simulink model "RB_KAIROS_BaseOnly"  (R2020b)
settings: Solver=ode4  StartTime=0.0  StopTime=t_end  FixedStep=Ts  RelTol=1e-3
values from neighbouring files (symbols this model uses):
  am = 0.3    [RB_KAIROS_ImpControl_OpSpace_BaseOnly.m]
  am_r = 0.3    [RB_KAIROS_ImpControl_OpSpace_BaseOnly.m]
  Jv = [1 0 0; 0 1 0; 0 0 0; 0 0 0; 0 0 0; 0 0 1;]    [RB_KAIROS_ImpControl_OpSpace_BaseOnly.m]
  Kc = diag(5*[1000,1000,0,0,0,1000])    [RB_KAIROS_ImpControl_OpSpace_BaseOnly.m]
  model_sample_time = 0.001    [RB_KAIROS_ImpControl_OpSpace_BaseOnly.m]
  q_dot_0 = zeros(10,1)    [RB_KAIROS_ImpControl_OpSpace_BaseOnly.m]
  T_i = T_W_V    [RB_KAIROS_ImpControl_OpSpace_BaseOnly.m]
  tau_ext = [0 0 0]    [RB_KAIROS_ImpControl_OpSpace_BaseOnly.m]
  v_SMU = 10    [RB_KAIROS_ImpControl_OpSpace_BaseOnly.m]
  vm = 0.6    [RB_KAIROS_ImpControl_OpSpace_BaseOnly.m]
  vm_r = 0.6    [RB_KAIROS_ImpControl_OpSpace_BaseOnly.m]
undefined symbols (not defined in the file or in its folder): DiscIntNeverNeededParam, magnitude, q_0, T_f
libraries: simulink x4, utils x4, transformations_lib x1
(part 2 of 16)

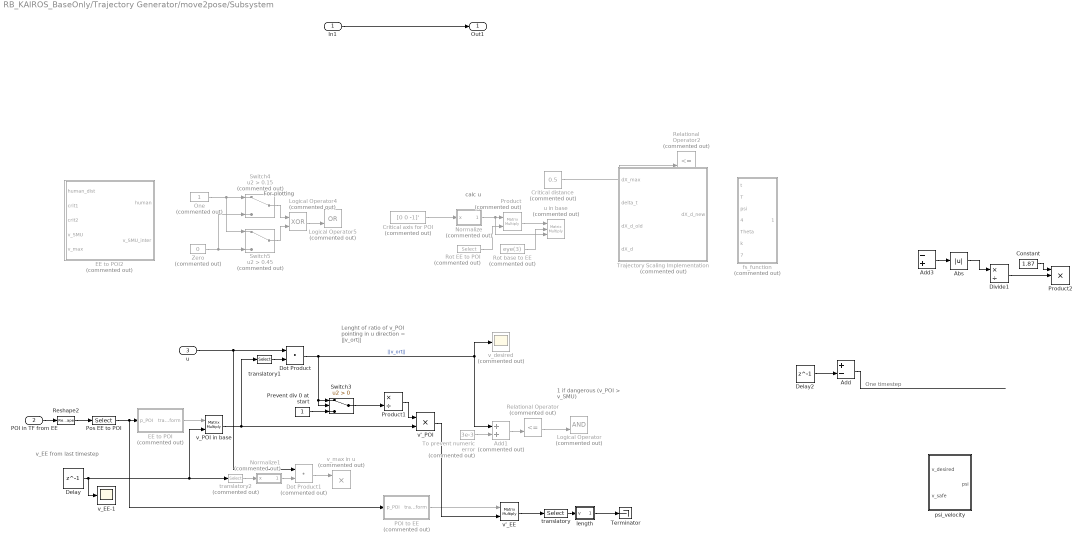
== system RB_KAIROS_BaseOnly/Trajectory Generator/move2pose/Subsystem ==
  note: calc u
  note: For plotting
  note: v_EE from last timestep
  note: 1 if dangerous
      | (v_POI > v_SMU)
  note: Lenght of ratio of v_POI
      | pointing in u direction
      | = ||v_ort||
  note: One timestep
  In1 : Inport
  POI in TF from EE : Inport  Port=2
  u : Inport  Port=3
  Abs : Abs
  Add : Sum  Inputs=+-
  Add1 : Sum  Commented=on
  Add3 : Sum  Inputs=-+
  Constant : Constant  Value=1.87
  Critical axis for POI : Constant  Commented=on  Value=[0 0 -1]'
  Critical distance : Constant  Commented=on  Value=0.5
  Delay : Delay  DelayLength=1
  Delay2 : Delay  DelayLength=1
  Divide1 : Product  Inputs=*/
  Dot Product : DotProduct  InputSameDT=on  OutDataTypeStr=Inherit: Inherit via internal rule
  Dot Product1 : DotProduct  Commented=on  InputSameDT=on  OutDataTypeStr=Inherit: Inherit via internal rule
  EE to POI : MATLAB Function  Commented=on  TreatAsAtomicUnit=on
  EE to POI2 : MATLAB Function  Commented=on  TreatAsAtomicUnit=on
  Logical Operator : Logic  Commented=on  AllPortsSameDT=off  OutDataTypeStr=boolean
  Logical Operator4 : Logic  Commented=on  Operator=XOR  AllPortsSameDT=off  OutDataTypeStr=boolean
  Logical Operator5 : Logic  Commented=on  Operator=OR  AllPortsSameDT=off  OutDataTypeStr=boolean
  Normalize : Subsystem  Commented=on
  Normalize1 : Subsystem  Commented=on
  One : Constant  Commented=on
  POI to EE : MATLAB Function  Commented=on  TreatAsAtomicUnit=on
  Pos EE to POI : Selector  NumberOfDimensions=2  InputPortWidth=7  IndexOptions=Index vector (dialog),Index vector (dialog)  Indices=[1:3],[4]  OutputSizes=1
  Prevent div 0 at start : Constant
  Product : Product  Commented=on  Multiplication=Matrix(*)
  Product1 : Product  Inputs=*/
  Product2 : Product  Inputs=3
  Relational Operator : RelationalOperator  Commented=on  Operator=<=  OutDataTypeStr=boolean  RndMeth=Simplest
  Relational Operator2 : RelationalOperator  Commented=on  Operator=<=  OutDataTypeStr=boolean  RndMeth=Simplest
  Reshape2 : Reshape  OutputDimensionality=Customize  OutputDimensions=[4,4]
  Rot EE to POI : Selector  Commented=on  NumberOfDimensions=2  InputPortWidth=7  IndexOptions=Index vector (dialog),Index vector (dialog)  Indices=[1:3],[1:3]  OutputSizes=1
  Rot base to EE : Constant  Commented=on  Value=eye(3)
  Switch3 : Switch  Criteria=u2 > Threshold
  Switch4 : Switch  Commented=on  Criteria=u2 > Threshold  Threshold=0.15
  Switch5 : Switch  Commented=on  Criteria=u2 > Threshold  Threshold=0.45
  Terminator : Terminator
  To prevent numeric error : Constant  Commented=on  Value=3e-3
  Trajectory Scaling Implementation : MATLAB Function  Commented=on  TreatAsAtomicUnit=on
  Zero : Constant  Commented=on  Value=0
  fs_function : MATLAB Function  Commented=on  TreatAsAtomicUnit=on
  length : Subsystem
  psi_velocity : MATLAB Function  TreatAsAtomicUnit=on
  translatory : Selector  InputPortWidth=6  IndexOptions=Index vector (dialog)  Indices=[1:3]  OutputSizes=1
  translatory1 : Selector  InputPortWidth=6  IndexOptions=Index vector (dialog)  Indices=[1:3]  OutputSizes=1
  translatory2 : Selector  Commented=on  InputPortWidth=6  IndexOptions=Index vector (dialog)  Indices=[1:3]  OutputSizes=1
  u in base : Product  Commented=on  Inputs=3  Multiplication=Matrix(*)
  v'_EE : Product  Multiplication=Matrix(*)
  v'_POI : Product
  v_EE-1 : Scope
  v_POI in base : Product  Multiplication=Matrix(*)
  v_desired : Scope  Commented=on
  v_max in u : Product  Commented=on
  Out1 : Outport  VectorParamsAs1DForOutWhenUnconnected=off
  wires:
  In1/1 -> Out1/1
  Critical axis for POI/1 -> Normalize/1(x)
  Rot EE to POI/1 -> Product/2
  Logical Operator4/1 -> Logical Operator5/2
  Product/1 -> u in base/1
  One/1 -> Switch4/1, Switch5/1
  Zero/1 -> Switch5/3, Switch4/3
  Switch4/1 -> Logical Operator4/1
  Switch5/1 -> Logical Operator4/2
  Normalize/1(x/||x||) -> u in base/3, Product/1
  Rot base to EE/1 -> u in base/2
  Critical distance/1 -> Relational Operator2/2
  Prevent div 0 at start/1 -> Switch3/3
  translatory2/1 -> Normalize1/1(x)
  Normalize1/1(x/||x||) -> Dot Product1/2
  ? -> Logical Operator/1
  ? -> v_max in u/2
  POI to EE/1(transform) -> v'_EE/1
  Add1/1 -> Relational Operator/2
  ? -> Product1/1
  v'_EE/1 -> translatory/1
  v'_POI/1 -> v'_EE/2
  EE to POI/1(transform) -> v_POI in base/1
  translatory/1 -> length/1(v)
  ? -> Relational Operator/1
  ? -> Delay/1
  v_POI in base/1 -> v'_POI/2, translatory1/1
  Dot Product1/1 -> v_max in u/1
  Delay/1 -> v_EE-1/1, v_POI in base/2, translatory2/1
  Dot Product/1 -> v_desired/1, Add1/1, Switch3/2, Switch3/1  "||v_ort||"
  translatory1/1 -> Dot Product/2
  Switch3/1 -> Product1/2
  Pos EE to POI/1 -> POI to EE/1(p_POI), EE to POI/1(p_POI)
  Reshape2/1 -> Pos EE to POI/1
  u/1 -> Dot Product/1, Dot Product1/1
  POI in TF from EE/1 -> Reshape2/1
  To prevent numeric error/1 -> Add1/2
  Product1/1 -> v'_POI/1
  length/1(|v|) -> Terminator/1
  Relational Operator/1 -> Logical Operator/2
  Delay2/1 -> Add/2
  ? -> Add/1
  ? -> Delay2/1
  Add/1 -> ?
  Abs/1 -> Divide1/1
  Constant/1 -> Product2/1
  Divide1/1 -> Product2/2
  Add3/1 -> Abs/1

== system RB_KAIROS_BaseOnly/CONTROLLER /Kinematics and Dynamics/Kinematics - error representation/Compute J_x_dot ==
  note: J_x_dot = R_D_W_aug*J_b_dot - R_D_W_aug*S(omega_d)_aug*J_b = R_D_W_aug*(J_b_dot - S(omega_d)_aug*J_b)
  J_b : Inport
  R_D_W_aug : Inport  Port=2
  x_dot_d : Inport  Port=3
  qv : Inport  Port=4
  qa : Inport  Port=5
  qv_dot : Inport  Port=6
  qa_dot : Inport  Port=7
  Add : Sum  Inputs=+-
  Augment matrix : MATLAB Function  TreatAsAtomicUnit=on
  MATLAB Function : MATLAB Function  TreatAsAtomicUnit=on
  MatrixMultiply : Product  Multiplication=Matrix(*)
  MatrixMultiply1 : Product  Multiplication=Matrix(*)
  S(omega) : MATLAB Function  TreatAsAtomicUnit=on
  Selector : Selector  InputPortWidth=6  IndexOptions=Index vector (dialog)  Indices=[4:6]  OutputSizes=1
  Selector1 : Selector  NumberOfDimensions=2  InputPortWidth=3  IndexOptions=Index vector (dialog),Index vector (dialog)  Indices=[1:6],[1:3]  OutputSizes=1,1
  J_x_dot : Outport
  wires:
  qv_dot/1 -> MATLAB Function/3(qv_dot)
  x_dot_d/1 -> Selector/1
  MatrixMultiply1/1 -> Add/2
  Add/1 -> MatrixMultiply/2
  MATLAB Function/1(J_dot) -> Selector1/1
  S(omega)/1(S) -> Augment matrix/1(M)
  Selector/1 -> S(omega)/1(v)
  qa/1 -> MATLAB Function/2(qa)
  MatrixMultiply/1 -> J_x_dot/1
  qv/1 -> MATLAB Function/1(qv)
  Augment matrix/1(M_aug) -> MatrixMultiply1/1
  qa_dot/1 -> MATLAB Function/4(qa_dot)
  J_b/1 -> MatrixMultiply1/2
  R_D_W_aug/1 -> MatrixMultiply/1
  Selector1/1 -> Add/1

== system RB_KAIROS_BaseOnly/Trajectory Generator/Subsystem1/Angle Axis Via Quaternions/Quaternion To Angle Axis ==
  eta : Inport
  epsilon : Inport  Port=2
  Divide : Product  Inputs=*/
  Gain : Gain  Gain=2
  Product : Product  RndMeth=Zero
  Saturation : Saturate  UpperLimit=1  LowerLimit=-1
  Sqrt : Sqrt  SaturateOnIntegerOverflow=on
  Subtract : Sum  Inputs=+-
  Switch1 : Switch  Criteria=u2 ~= 0
  Trigonometric Function : Trigonometry  Operator=acos
  dummy axis : Constant  Value=[1,0,0]
  one : Constant
  angle : Outport  VectorParamsAs1DForOutWhenUnconnected=off
  axis : Outport  Port=2  VectorParamsAs1DForOutWhenUnconnected=off
  wires:
  Divide/1 -> Switch1/1
  Switch1/1 -> axis/1
  dummy axis/1 -> Switch1/3
  Gain/1 -> Switch1/2, angle/1
  epsilon/1 -> Divide/1
  Trigonometric Function/1 -> Gain/1
  eta/1 -> Saturation/1
  Subtract/1 -> Sqrt/1
  one/1 -> Subtract/1
  Product/1 -> Subtract/2
  Sqrt/1 -> Divide/2
  Saturation/1 -> Trigonometric Function/1, Product/1, Product/2

== system RB_KAIROS_BaseOnly/Trajectory Generator/Subsystem1/Normalize/length ==
  v : Inport
  Abs1 : Abs
  Add : Sum  Inputs=+
  Math Function : Math  Operator=magnitude^2  SignedPower=on  SaturateOnIntegerOverflow=on
  Sqrt : Sqrt  Operator=signedSqrt  SaturateOnIntegerOverflow=on
  |v| : Outport  VectorParamsAs1DForOutWhenUnconnected=off
  wires:
  Math Function/1 -> Add/1
  Add/1 -> Sqrt/1
  v/1 -> Math Function/1
  Abs1/1 -> |v|/1
  Sqrt/1 -> Abs1/1

== system RB_KAIROS_BaseOnly/Trajectory Generator/move2pose/Cartesian_ipol2/rotation ==
  t : Inport
  phi_0 : Inport  Port=2
  dphi_0 : Inport  Port=3
  phi_f : Inport  Port=4
  dphi_max : Inport  Port=5
  ddphi_max : Inport  Port=6
  T_scale : Inport  Port=7
  interpoly : Inport  Port=8
  Abs1 : Abs
  Compare To Constant : simulink/Logic and Bit Operations/Compare To Constant  relop=<=  const=1e-9  OutDataTypeStr=boolean
  Data Type Conversion : DataTypeConversion  OutDataTypeStr=boolean
  Embedded MATLAB Function1 : MATLAB Function  TreatAsAtomicUnit=on
  Logical Operator2 : Logic  Operator=OR  AllPortsSameDT=off  OutDataTypeStr=boolean
  Subtract1 : Sum  Inputs=-+
  T7 : Terminator
  phi_d : Outport  VectorParamsAs1DForOutWhenUnconnected=off
  d_phi_d : Outport  Port=2  VectorParamsAs1DForOutWhenUnconnected=off
  ipol_finished : Outport  Port=3  VectorParamsAs1DForOutWhenUnconnected=off
  wires:
  ddphi_max/1 -> Embedded MATLAB Function1/6(am)
  dphi_max/1 -> Embedded MATLAB Function1/5(vm)
  dphi_0/1 -> Embedded MATLAB Function1/3(v0)
  phi_0/1 -> Embedded MATLAB Function1/2(s0)
  t/1 -> Embedded MATLAB Function1/1(t)
  Embedded MATLAB Function1/3(ddqd) -> T7/1
  interpoly/1 -> Embedded MATLAB Function1/8(interpoly)
  T_scale/1 -> Embedded MATLAB Function1/7(T_scale)
  Compare To Constant/1 -> Logical Operator2/2
  Subtract1/1 -> Abs1/1
  Abs1/1 -> Compare To Constant/1
  Logical Operator2/1 -> ipol_finished/1
  Embedded MATLAB Function1/4(ipol_finished) -> Data Type Conversion/1
  Data Type Conversion/1 -> Logical Operator2/1
  phi_f/1 -> Subtract1/2, Embedded MATLAB Function1/4(sf)
  Embedded MATLAB Function1/2(dqd) -> d_phi_d/1
  Embedded MATLAB Function1/1(qd) -> phi_d/1, Subtract1/1

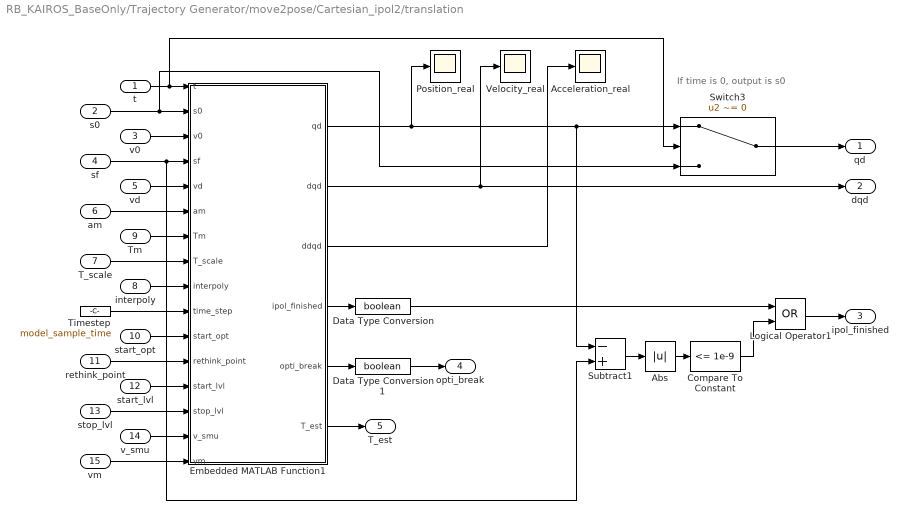
== system RB_KAIROS_BaseOnly/Trajectory Generator/move2pose/Cartesian_ipol2/translation ==
  note: If time is 0, output is s0
  t : Inport
  s0 : Inport  Port=2
  v0 : Inport  Port=3
  sf : Inport  Port=4
  vd : Inport  Port=5
  am : Inport  Port=6
  T_scale : Inport  Port=7
  interpoly : Inport  Port=8
  Tm : Inport  Port=9
  start_opt : Inport  Port=10
  rethink_point : Inport  Port=11
  start_lvl : Inport  Port=12
  stop_lvl : Inport  Port=13
  v_smu : Inport  Port=14
  vm : Inport  Port=15
  Abs : Abs
  Acceleration_real : Scope
  Compare To Constant : simulink/Logic and Bit Operations/Compare To Constant  relop=<=  const=1e-9  OutDataTypeStr=boolean
  Data Type Conversion : DataTypeConversion  OutDataTypeStr=boolean
  Data Type Conversion1 : DataTypeConversion  OutDataTypeStr=boolean
  Embedded MATLAB Function1 : MATLAB Function  TreatAsAtomicUnit=on
  Logical Operator1 : Logic  Operator=OR  AllPortsSameDT=off  OutDataTypeStr=boolean
  Position_real : Scope
  Subtract1 : Sum  Inputs=-+
  Switch3 : Switch  Criteria=u2 ~= 0
  Timestep : Constant  Value=model_sample_time
  Velocity_real : Scope
  qd : Outport  VectorParamsAs1DForOutWhenUnconnected=off
  dqd : Outport  Port=2  VectorParamsAs1DForOutWhenUnconnected=off
  ipol_finished : Outport  Port=3  VectorParamsAs1DForOutWhenUnconnected=off
  opti_break : Outport  Port=4  VectorParamsAs1DForOutWhenUnconnected=off
  T_est : Outport  Port=5  VectorParamsAs1DForOutWhenUnconnected=off
  wires:
  Switch3/1 -> qd/1
  Logical Operator1/1 -> ipol_finished/1
  Embedded MATLAB Function1/2(dqd) -> Velocity_real/1, dqd/1
  Embedded MATLAB Function1/1(qd) -> Switch3/1, Subtract1/1, Position_real/1
  s0/1 -> Embedded MATLAB Function1/2(s0), Switch3/3
  t/1 -> Switch3/2, Embedded MATLAB Function1/1(t)
  am/1 -> Embedded MATLAB Function1/6(am)
  vd/1 -> Embedded MATLAB Function1/5(vd)
  v0/1 -> Embedded MATLAB Function1/3(v0)
  Subtract1/1 -> Abs/1
  Compare To Constant/1 -> Logical Operator1/2
  Abs/1 -> Compare To Constant/1
  Embedded MATLAB Function1/3(ddqd) -> Acceleration_real/1
  T_scale/1 -> Embedded MATLAB Function1/8(T_scale)
  interpoly/1 -> Embedded MATLAB Function1/9(interpoly)
  Embedded MATLAB Function1/4(ipol_finished) -> Data Type Conversion/1
  Data Type Conversion/1 -> Logical Operator1/1
  Timestep/1 -> Embedded MATLAB Function1/10(time_step)
  Tm/1 -> Embedded MATLAB Function1/7(Tm)
  Embedded MATLAB Function1/5(opti_break) -> Data Type Conversion1/1
  Data Type Conversion1/1 -> opti_break/1
  Embedded MATLAB Function1/6(T_est) -> T_est/1
  start_opt/1 -> Embedded MATLAB Function1/11(start_opt)
  rethink_point/1 -> Embedded MATLAB Function1/12(rethink_point)
  start_lvl/1 -> Embedded MATLAB Function1/13(start_lvl)
  stop_lvl/1 -> Embedded MATLAB Function1/14(stop_lvl)
  v_smu/1 -> Embedded MATLAB Function1/15(v_smu)
  vm/1 -> Embedded MATLAB Function1/16(vm)
  sf/1 -> Subtract1/2, Embedded MATLAB Function1/4(sf)

== system RB_KAIROS_BaseOnly/Trajectory Generator/move2pose/Subsystem/Normalize ==
  x : Inport
  Divide : Product  Inputs=*/
  Switch : Switch  Criteria=u2 > Threshold
  length : Subsystem
  one : Constant
  x/||x|| : Outport  VectorParamsAs1DForOutWhenUnconnected=off
  wires:
  x/1 -> Divide/1, length/1(v)
  Divide/1 -> x/||x||/1
  one/1 -> Switch/3
  length/1(|v|) -> Switch/2, Switch/1
  Switch/1 -> Divide/2

== system RB_KAIROS_BaseOnly/Trajectory Generator/move2pose/Subsystem/Normalize1 ==
  x : Inport
  Divide : Product  Inputs=*/
  Switch : Switch  Criteria=u2 > Threshold
  length : Subsystem
  one : Constant
  x/||x|| : Outport  VectorParamsAs1DForOutWhenUnconnected=off
  wires:
  x/1 -> Divide/1, length/1(v)
  Divide/1 -> x/||x||/1
  one/1 -> Switch/3
  length/1(|v|) -> Switch/2, Switch/1
  Switch/1 -> Divide/2

== system RB_KAIROS_BaseOnly/Trajectory Generator/move2pose/Subsystem/length ==
  v : Inport
  Abs1 : Abs
  Add : Sum  Inputs=+
  Math Function : Math  Operator=magnitude^2  SignedPower=on  SaturateOnIntegerOverflow=on
  Sqrt : Sqrt  Operator=signedSqrt  SaturateOnIntegerOverflow=on
  |v| : Outport  VectorParamsAs1DForOutWhenUnconnected=off
  wires:
  Math Function/1 -> Add/1
  Add/1 -> Sqrt/1
  v/1 -> Math Function/1
  Abs1/1 -> |v|/1
  Sqrt/1 -> Abs1/1

== system RB_KAIROS_BaseOnly/Trajectory Generator/move2pose/Subsystem/Normalize/length ==
  v : Inport
  Add : Sum  Inputs=+
  Math Function : Math  Operator=magnitude^2  SignedPower=on  SaturateOnIntegerOverflow=on
  Math Function1 : Math  Operator=sqrt  SignedPower=on  SaturateOnIntegerOverflow=on
  |v| : Outport  VectorParamsAs1DForOutWhenUnconnected=off
  wires:
  Math Function/1 -> Add/1
  Add/1 -> Math Function1/1
  v/1 -> Math Function/1
  Math Function1/1 -> |v|/1

== system RB_KAIROS_BaseOnly/Trajectory Generator/move2pose/Subsystem/Normalize1/length ==
  v : Inport
  Abs1 : Abs
  Add : Sum  Inputs=+
  Math Function : Math  Operator=magnitude^2  SignedPower=on  SaturateOnIntegerOverflow=on
  Sqrt : Sqrt  Operator=signedSqrt  SaturateOnIntegerOverflow=on
  |v| : Outport  VectorParamsAs1DForOutWhenUnconnected=off
  wires:
  Math Function/1 -> Add/1
  Add/1 -> Sqrt/1
  v/1 -> Math Function/1
  Abs1/1 -> |v|/1
  Sqrt/1 -> Abs1/1

== matlab function RB_KAIROS_BaseOnly/CONTROLLER /Kinematics and Dynamics/Compute quantities ==
  data: M input; C input; Lambda output; mu output; J_x_T output; J_x input; J_x_d input; J_x_i output
function [Lambda, mu, J_x_T, J_x_i] = configuration_to_cartesian(M,C,J_x,J_x_d)

%Converts Mass Matrix, Coriolis/Centrifugal Matrix to Cartesian space
%representation

%M_i = inv(M);

%For redundant robots, it is not possible to direclty get the Mass Matrix
%in the cartesia space, thus a "pseudo Mass Matrix" is provided (this is 
%valid also for non-redundant robots):
J_x
Lambda_i = J_x/M*J_x'

%Here pinv is used for ensuring an inverse also in case of singular
%matrices. This is particularly useful when the selected Jacobian is
%considering only the arm or the vehicle.
Lambda = pinv(Lambda_i)

%Dynamically consistent pseudo-inverse:
J_x_i = M\J_x'*Lambda; 

%Cartesian Coriolis/Centrifugal Matrix
mu = J_x_i'*(C-M*J_x_i*J_x_d)*J_x_i;

%transpose of the Jacobian
J_x_T = J_x';
